simulink model "traditionpid"  (Simulink 8.7)
settings: Solver=VariableStepAuto  StartTime=0.0  StopTime=10  RelTol=1e-3
values from neighbouring files (symbols this model uses):
  M = 2.5    [workspace_data.mat]
  miu = 4.6    [workspace_data.mat]
settings Model: Creator=Administrator  LastModifiedBy=Administrator
settings DataIOCC: LimitDataPoints=off  SaveFormat=Dataset
settings DebuggingCC: UnderspecifiedInitializationDetection=Simplified  MergeDetectMultiDrivingBlocksExec=error
settings HardwareCC: ProdBitPerPointer=64  ProdLargestAtomicFloat=Float  ProdIntDivRoundTo=Zero  ProdEndianess=LittleEndian  ProdWordSize=64  ProdHWDeviceType=Intel->x86-64 (Windows64)
settings ModelReferenceCC: PropagateSignalLabelsOutOfModel=on
settings ConfigComp: CovModelRefEnable=off

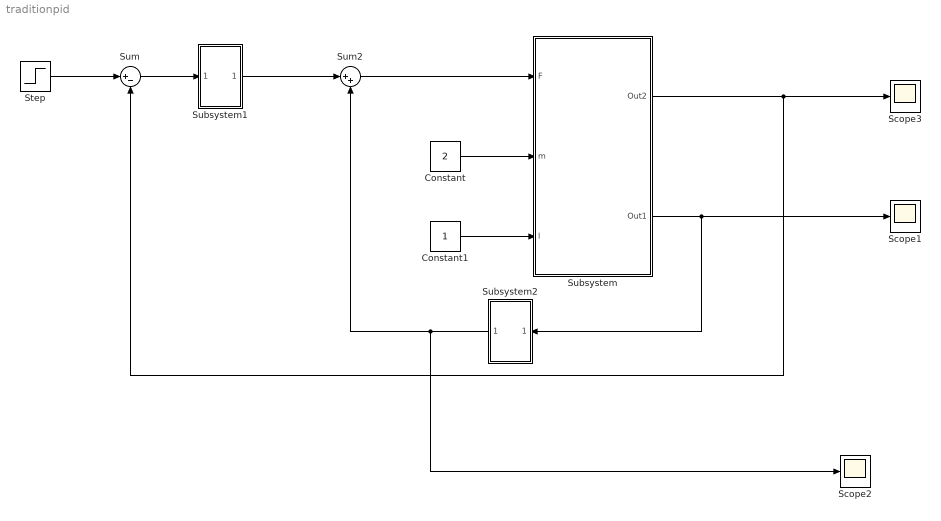
== system traditionpid ==
  Constant : Constant  Value=2
  Constant1 : Constant
  Scope1 : Scope
  Scope2 : Scope
  Scope3 : Scope
  Step : Step  SampleTime=0
  Subsystem : Subsystem
  Subsystem1 : Subsystem
  Subsystem2 : Subsystem
  Sum : Sum  Inputs=|+-
  Sum2 : Sum  Inputs=|++
  wires:
  Step/1 -> Sum/1
  Sum/1 -> Subsystem1/1(In1)
  Constant/1 -> Subsystem/2(m)
  Constant1/1 -> Subsystem/3(l)
  Sum2/1 -> Subsystem/1(F)
  Subsystem/1(Out2) -> Sum/2, Scope3/1
  Subsystem/2(Out1) -> Subsystem2/1(In1), Scope1/1
  Subsystem2/1(Out1) -> Scope2/1, Sum2/2
  Subsystem1/1(Out1) -> Sum2/1

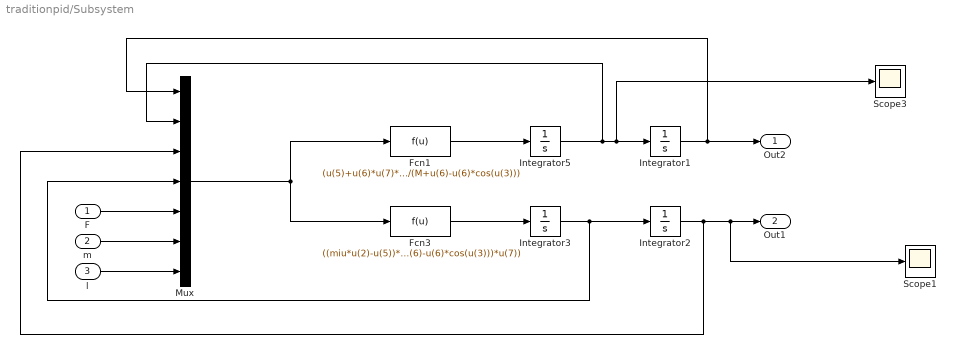
== system traditionpid/Subsystem ==
  F : Inport
  m : Inport  Port=2
  l : Inport  Port=3
  Fcn1 : Fcn  Expr=(u(5)+u(6)*u(7)*u(4)*u(4)*sin(u(3))+9.8*u(6)*sin(u(3))-miu*u(2))/(M+u(6)-u(6)*cos(u(3)))
  Fcn3 : Fcn  Expr=((miu*u(2)-u(5))*u(7)*cos(u(3))-(u(7)*u(7)*u(4)*u(4)+9.8*u(7)*9.8)*u(6)*sin(u(3))*cos(u(3))-(M+u(6))*9.8*sin(u(3)))/((M+u(6)-u(6)*cos(u(3)))*u(7))
  Integrator{1..3,5} (4 alike) : Integrator
  Mux : Mux  Inputs=7
  Scope1 : Scope
  Scope3 : Scope
  Out2 : Outport
  Out1 : Outport  Port=2
  wires:
  Integrator1/1 -> Out2/1, Mux/1
  l/1 -> Mux/7
  Fcn3/1 -> Integrator3/1
  F/1 -> Mux/5
  Integrator3/1 -> Mux/4, Integrator2/1
  Integrator5/1 -> Mux/2, Scope3/1, Integrator1/1
  m/1 -> Mux/6
  Mux/1 -> Fcn3/1, Fcn1/1
  Fcn1/1 -> Integrator5/1
  Integrator2/1 -> Scope1/1, Out1/1, Mux/3

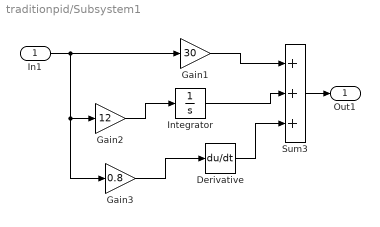
== system traditionpid/Subsystem1 ==
  In1 : Inport
  Derivative : Derivative
  Gain1 : Gain  Gain=30
  Gain2 : Gain  Gain=12
  Gain3 : Gain  Gain=0.8
  Integrator : Integrator
  Sum3 : Sum  Inputs=+++
  Out1 : Outport
  wires:
  Gain1/1 -> Sum3/1
  Integrator/1 -> Sum3/2
  Derivative/1 -> Sum3/3
  Gain3/1 -> Derivative/1
  Gain2/1 -> Integrator/1
  In1/1 -> Gain1/1, Gain2/1, Gain3/1
  Sum3/1 -> Out1/1

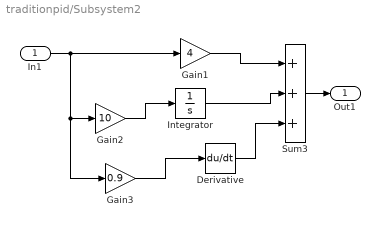
== system traditionpid/Subsystem2 ==
  In1 : Inport
  Derivative : Derivative
  Gain1 : Gain  Gain=4
  Gain2 : Gain  Gain=10
  Gain3 : Gain  Gain=0.9
  Integrator : Integrator
  Sum3 : Sum  Inputs=+++
  Out1 : Outport
  wires:
  Gain1/1 -> Sum3/1
  Integrator/1 -> Sum3/2
  Derivative/1 -> Sum3/3
  Gain3/1 -> Derivative/1
  Gain2/1 -> Integrator/1
  In1/1 -> Gain1/1, Gain2/1, Gain3/1
  Sum3/1 -> Out1/1
